simulink model "DualMotorElectricVehicle_full_Accel_full_Brake"  (R2023b)
settings: Solver=FixedStepAuto  StartTime=0.0  StopTime=300  FixedStep=0.01  RelTol=1e-3
values from neighbouring files (symbols this model uses):
  Af = 2.4    [DualMotorElectricVehicle.m]    (also in DualMotorElectricVehicle_Parameter.m)
  Cd = 0.24    [DualMotorElectricVehicle.m]    (also in DualMotorElectricVehicle_Parameter.m)
  eff_map_f = [ 81.3 81.3 82.2 82.0 81.5 81.2 80.4 79.3 80.1 76.8 74.3 73.5 72.0 71.6 70.0 71.1 ... (first row only)    [DualMotorElectricVehicle.m]    (also in DualMotorElectricVehicle_Parameter.m)
  eff_map_r = [ 36.6 36.6 36.6 36.6 36.6 36.6 36.6 36.6 36.6 36.6 36.6 36.6 36.6 36.6 36.6 36.6 36.6 36.6 36.6 36.6 36.6 36.6 36.6 36.6 36.6 36.6 36.6 36.6 36.6 36.6 36.6 36.6 36.6 36.6 36.6 36.6 36.6 36.6 36.6 36.6 36.6 ... (first row only)    [DualMotorElectricVehicle.m]    (also in DualMotorElectricVehicle_Parameter.m)
  eff_spd_f = [0 105 209 314 419 524 628 733 838 943 1047 1152 1257 1361]*30/pi    [DualMotorElectricVehicle.m]    (also in DualMotorElectricVehicle_Parameter.m)
  eff_spd_r = [0 300 500 700 900 1100 1300 1500 1700 1900 2100 2300 2500 2700 3000 3400 3800 4200 4600 5000 5400 5800 6000]    [DualMotorElectricVehicle.m]    (also in DualMotorElectricVehicle_Parameter.m)
  eff_trq_f = [0.0 13.6 27.1 40.7 54.2 67.8 81.4 94.9 108.5 122.0 135.6 149.2 162.7 176.3 189.8 203.4]    [DualMotorElectricVehicle.m]    (also in DualMotorElectricVehicle_Parameter.m)
  eff_trq_r = [0:5:200]*125/200    [DualMotorElectricVehicle.m]    (also in DualMotorElectricVehicle_Parameter.m)
  f_roll = 0.015    [DualMotorElectricVehicle.m]    (also in DualMotorElectricVehicle_Parameter.m)
  g = 9.81    [DualMotorElectricVehicle.m]    (also in DualMotorElectricVehicle_Parameter.m)
  G_final = 8    [DualMotorElectricVehicle.m]    (also in DualMotorElectricVehicle_Parameter.m)
  M_veh = 2000    [DualMotorElectricVehicle.m]    (also in DualMotorElectricVehicle_Parameter.m)
  Q_bat = 28    [DualMotorElectricVehicle.m]    (also in DualMotorElectricVehicle_Parameter.m)
  R_final = 4    [DualMotorElectricVehicle.m]    (also in DualMotorElectricVehicle_Parameter.m)
  R_int = 0.2811    [DualMotorElectricVehicle.m]    (also in DualMotorElectricVehicle_Parameter.m)
  r_tire = 0.35    [DualMotorElectricVehicle.m]    (also in DualMotorElectricVehicle_Parameter.m)
  rho = 1.16    [DualMotorElectricVehicle.m]    (also in DualMotorElectricVehicle_Parameter.m)
  SOC_init = 0.9    [DualMotorElectricVehicle.m]    (also in DualMotorElectricVehicle_Parameter.m = 0.8)
  SOC_min = 0.2    [DualMotorElectricVehicle.m]    (also in DualMotorElectricVehicle_Parameter.m = 0.4)
  tau_f = 0.05    [DualMotorElectricVehicle_Parameter.m]
  tau_m = 0.015    [DualMotorElectricVehicle_Parameter.m]
  theta = 0    [DualMotorElectricVehicle.m]    (also in DualMotorElectricVehicle_Parameter.m)
  Tm_max_spd_f = [0 300 419 524 628 733 838 943 1047 1152 1257 1361 1461 1561]*30/pi    [DualMotorElectricVehicle.m]    (also in DualMotorElectricVehicle_Parameter.m)
  Tm_max_spd_r = [0 1230 1300 1500:500:5500 5800 6000]    [DualMotorElectricVehicle.m]    (also in DualMotorElectricVehicle_Parameter.m)
  Tm_max_trq_f = [203 203 193 156 129 111 98 85 79 72 65 60 0 0]    [DualMotorElectricVehicle.m]    (also in DualMotorElectricVehicle_Parameter.m)
  Tm_max_trq_r = [125 125 117.53 101.86 76.39 61.12 50.93 43.65 38.20 33.95 30.56 27.78 0 0]    [DualMotorElectricVehicle.m]    (also in DualMotorElectricVehicle_Parameter.m)
  VOC_map = No_cell * [3.19, 3.40, 3.47, 3.59, 3.62, 3.65, 3.69, 3.74, 3.82, 3.89, 3.96]    [DualMotorElectricVehicle.m]    (also in DualMotorElectricVehicle_Parameter.m)
  VOC_SOC = [0, 0.1, 0.2, 0.3, 0.4, 0.5, 0.6 0.7, 0.8, 0.9, 1]    [DualMotorElectricVehicle.m]    (also in DualMotorElectricVehicle_Parameter.m)
  Vt_init = 311    [DualMotorElectricVehicle.m]    (also in DualMotorElectricVehicle_Parameter.m)
libraries: SignalEditorBlockLib x2
settings Model: Creator=김준현  LastModifiedBy=김준현

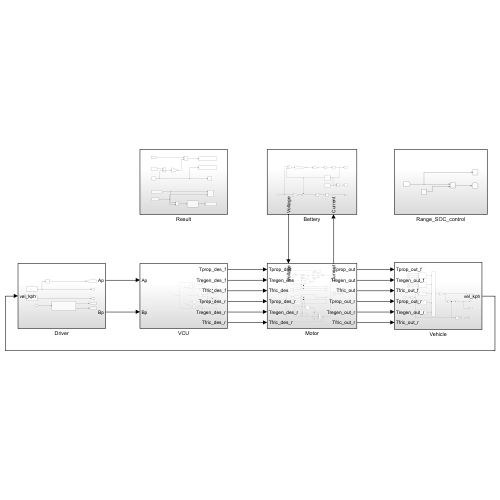
[thumbnail: Simulink's stored preview of the top-level diagram]
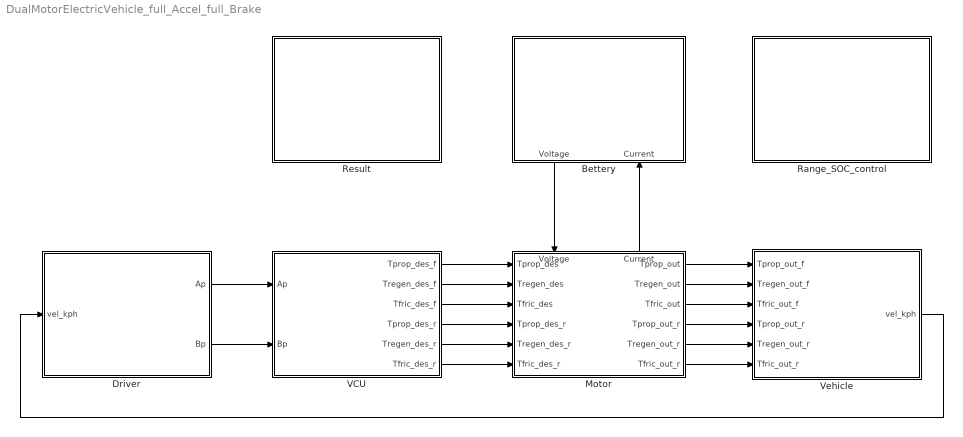
== system DualMotorElectricVehicle_full_Accel_full_Brake ==
  Bettery : Subsystem
      settings: PortSchema="{\"entries\":[{\"content\":{\"sides\":[{\"content\":{},\"type\":\"ConnectorPlacement.EquallySpacedRectSide\",\"uuid\":\"4f8bbb1a-fa5a-421b-ae69-e0b44ed86b01\"},{\"content\":{\"side\":\"RIGHT\"},\"type\":\"ConnectorPlacement.EquallySpacedRectSide\",\"uuid\":\"64d9ef76-34ca-4a4b-a58c-5ada3c393ba3\"},{\"content\":{\"side\":\"TOP\"},\"type\":\"ConnectorPlacement.EquallySpacedRectSide\",\"uuid\":\"8e5f7bf2-c6ce-4b8d-bfcf-b49871de395a\"},{\"content\":{\"connectorIds\":[\"Out1\",\"In1\"],\"side\":\"BOTTOM\"},\"type\":\"ConnectorPlacement.EquallySpacedRectSide\",\"uuid\":\"99b45dde-6c00-4863-951a-4b4ae2772398\"}]},\"type\":\"ConnectorPlacement.EquallySpacedConnector\",\"uuid\":\"2f749249-48ed-4409-ad27-f14061cdc912\"}],\"packageUris\":[\"http://schema.mathworks.com/mf0/Connector/R2020b\"],\"version\":\"1.0\"}"
  Driver : Subsystem
  Motor : Subsystem
      settings: PortSchema="{\"entries\":[{\"content\":{\"sides\":[{\"content\":{\"connectorIds\":[\"In1\",\"In2\",\"In3\",\"In4\",\"In5\",\"In6\"]},\"type\":\"ConnectorPlacement.EquallySpacedRectSide\",\"uuid\":\"a94dc67e-5088-4d58-a4ca-eb86600f42a3\"},{\"content\":{\"connectorIds\":[\"Out1\",\"Out2\",\"Out3\",\"Out4\",\"Out5\",\"Out6\"],\"side\":\"RIGHT\"},\"type\":\"ConnectorPlacement.EquallySpacedRectSide\",\"uuid\":\"bb581995-727b-4bbc-b281-e0daf5ac58fc\"},{\"content\":{\"connectorIds\":[\"In7\",\"Out7\"],\"side\":\"TOP\"},\"type\":\"ConnectorPlacement.EquallySpacedRectSide\",\"uuid\":\"7ea9d0e6-8443-414c-bafd-4c6fdb6eb2aa\"}]},\"type\":\"ConnectorPlacement.EquallySpacedConnector\",\"uuid\":\"c06b5305-48a4-41e7-b050-c7ca45c72c8b\"}],\"packageUris\":[\"http://schema.mathworks.com/mf0/Connector/R2020b\"],\"version\":\"1.0\"}"
  Range_SOC_control : Subsystem
  Result : Subsystem
  VCU : Subsystem
  Vehicle : Subsystem
  wires:
  Driver/1(Ap) -> VCU/1(Ap)
  Driver/2(Bp) -> VCU/2(Bp)
  VCU/1(Tprop_des_f) -> Motor/1(Tprop_des)
  VCU/2(Tregen_des_f) -> Motor/2(Tregen_des)
  VCU/3(Tfric_des_f) -> Motor/3(Tfric_des)
  Bettery/1(Voltage) -> Motor/7(Voltage)
  Motor/7(Current) -> Bettery/1(Current)
  Motor/1(Tprop_out) -> Vehicle/1(Tprop_out_f)
  Motor/2(Tregen_out) -> Vehicle/2(Tregen_out_f)
  Motor/3(Tfric_out) -> Vehicle/3(Tfric_out_f)
  Vehicle/1(vel_kph) -> Driver/1(vel_kph)
  VCU/4(Tprop_des_r) -> Motor/4(Tprop_des_r)
  VCU/5(Tregen_des_r) -> Motor/5(Tregen_des_r)
  VCU/6(Tfric_des_r) -> Motor/6(Tfric_des_r)
  Motor/4(Tprop_out_r) -> Vehicle/4(Tprop_out_r)
  Motor/5(Tregen_out_r) -> Vehicle/5(Tregen_out_r)
  Motor/6(Tfric_out_r) -> Vehicle/6(Tfric_out_r)

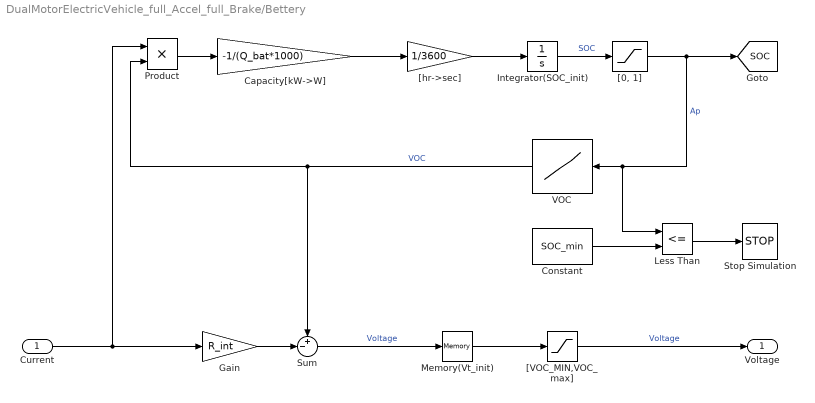
== system DualMotorElectricVehicle_full_Accel_full_Brake/Bettery ==
  Current : Inport
  Capacity[kW->W] : Gain  Gain=-1/(Q_bat*1000)
  Constant : Constant  Value=SOC_min
  Gain : Gain  Gain=R_int
  Integrator(SOC_init) : Integrator  InitialCondition=SOC_init
  Less Than : RelationalOperator  Operator=<=  OutDataTypeStr=boolean  RndMeth=Simplest  InputSameDT=off
  Memory(Vt_init) : Memory  InitialCondition=Vt_init
  Product : Product
  Stop Simulation : Stop
  Sum : Sum  Inputs=+-|
  VOC : Lookup_n-D  NumberOfTableDimensions=1  BreakpointsForDimension1=VOC_SOC  Table=VOC_map  InternalRulePriority=Speed  RndMeth=Simplest
  "[0, 1]" : Saturate  UpperLimit=1  LowerLimit=0
  "[VOC_MIN,VOC_max]" : Saturate  UpperLimit=max(VOC_map)  LowerLimit=min(VOC_map)
  "[hr->sec]" : Gain  Gain=1/3600
  Voltage : Outport
  tag scope: SOC=global
  wires:
  Current/1 -> Gain/1, Product/1
  VOC/1 -> Sum/1, Product/2  "VOC"
  Product/1 -> Capacity[kW->W]/1
  Capacity[kW->W]/1 -> "[hr->sec]"/1
  "[hr->sec]"/1 -> Integrator(SOC_init)/1
  Integrator(SOC_init)/1 -> "[0, 1]"/1  "SOC"
  Gain/1 -> Sum/2
  Sum/1 -> Memory(Vt_init)/1  "Voltage"
  "[VOC_MIN,VOC_max]"/1 -> Voltage/1  "Voltage"
  Memory(Vt_init)/1 -> "[VOC_MIN,VOC_max]"/1
  Less Than/1 -> Stop Simulation/1
  Constant/1 -> Less Than/2
  "[0, 1]"/1 -> [SOC], Less Than/1, VOC/1  "Ap"

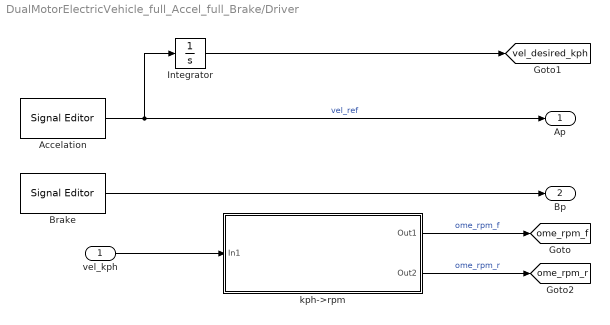
== system DualMotorElectricVehicle_full_Accel_full_Brake/Driver ==
  vel_kph : Inport
  Accelation : SignalEditorBlockLib/Signal Editor  FileName=AP.mat  ActiveScenario=Scenario  ActiveSignal=Step  IsBus=off  OutputBusObjectStr=Bus: BusObject  SampleTime=0  Interpolate=off  ZeroCross=off  OutputAfterFinalValue=Setting to zero  Unit=inherit  PreserveSignalName=on  ApplySigPropsToAllScenarios=on  ApplySigPropsToAllSignals=off
  Brake : SignalEditorBlockLib/Signal Editor  FileName=BP.mat  ActiveScenario=Scenario  ActiveSignal=Signal 1  IsBus=off  OutputBusObjectStr=Bus: BusObject  SampleTime=0  Interpolate=off  ZeroCross=off  OutputAfterFinalValue=Setting to zero  Unit=inherit  PreserveSignalName=on  ApplySigPropsToAllScenarios=on  ApplySigPropsToAllSignals=off
  Integrator : Integrator
  kph->rpm : Subsystem
  Ap : Outport
  Bp : Outport  Port=2
  tag scope: ome_rpm_f=global, ome_rpm_r=global, vel_desired_kph=global
  wires:
  kph->rpm/1(Out1) -> [ome_rpm_f]  "ome_rpm_f"
  vel_kph/1 -> kph->rpm/1(In1)
  Accelation/1 -> Ap/1, Integrator/1  "vel_ref"
  Integrator/1 -> [vel_desired_kph]
  Brake/1 -> Bp/1
  kph->rpm/2(Out2) -> [ome_rpm_r]  "ome_rpm_r"

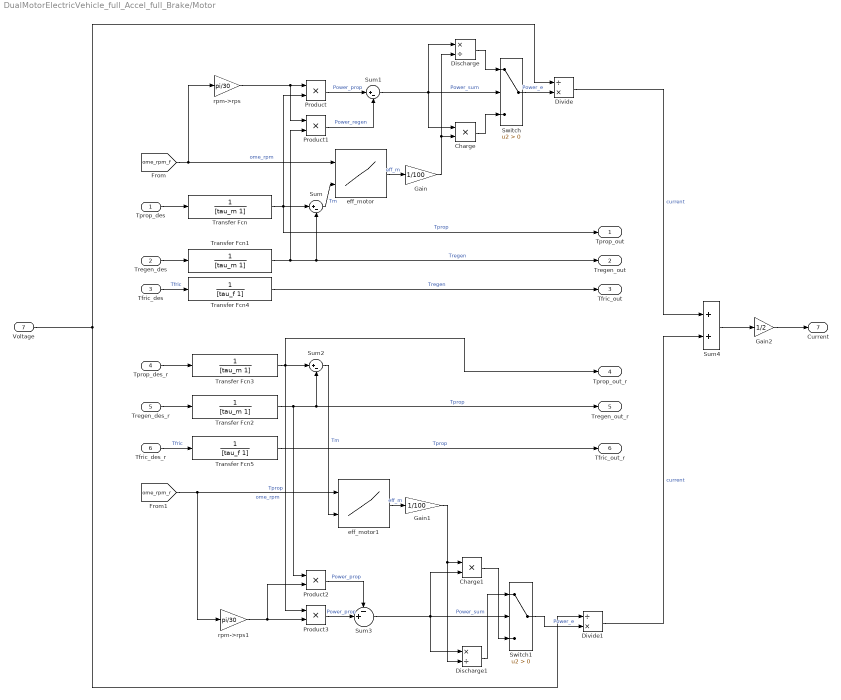
== system DualMotorElectricVehicle_full_Accel_full_Brake/Motor ==
  Tprop_des : Inport
  Tregen_des : Inport  Port=2
  Tfric_des : Inport  Port=3
  Tprop_des_r : Inport  Port=4
  Tregen_des_r : Inport  Port=5
  Tfric_des_r : Inport  Port=6
  Voltage : Inport  Port=7
  Charge : Product
  Charge1 : Product
  Discharge : Product  Inputs=*/
  Discharge1 : Product  Inputs=*/
  Divide : Product  Inputs=/*
  Divide1 : Product  Inputs=/*
  Gain : Gain  Gain=1/100
  Gain1 : Gain  Gain=1/100
  Gain2 : Gain  Gain=1/2
  Product{,1..3} (4 alike) : Product
  Sum : Sum  Inputs=|+-
  Sum1 : Sum  Inputs=|+-
  Sum2 : Sum  Inputs=|+-
  Sum3 : Sum  Inputs=-+|
  Sum4 : Sum
  Switch : Switch  Criteria=u2 > Threshold  SaturateOnIntegerOverflow=off  InputSameDT=off
  Switch1 : Switch  Criteria=u2 > Threshold  SaturateOnIntegerOverflow=off  InputSameDT=off
  Transfer Fcn{,1..3} (4 alike) : TransferFcn  Denominator=[tau_m 1]
  Transfer Fcn4 : TransferFcn  Denominator=[tau_f 1]
  Transfer Fcn5 : TransferFcn  Denominator=[tau_f 1]
  eff_motor : Lookup_n-D  BreakpointsForDimension1=eff_spd_f  BreakpointsForDimension2=eff_trq_f  Table=eff_map_f  InternalRulePriority=Speed  RndMeth=Simplest
      settings: InputPortMap=u0,u1
  eff_motor1 : Lookup_n-D  BreakpointsForDimension1=eff_spd_r  BreakpointsForDimension2=eff_trq_r  Table=eff_map_r  InternalRulePriority=Speed  RndMeth=Simplest
      settings: InputPortMap=u0,u1
  rpm->rps : Gain  Gain=pi/30
  rpm->rps1 : Gain  Gain=pi/30
  Tprop_out : Outport
  Tregen_out : Outport  Port=2
  Tfric_out : Outport  Port=3
  Tprop_out_r : Outport  Port=4
  Tregen_out_r : Outport  Port=5
  Tfric_out_r : Outport  Port=6
  Current : Outport  Port=7
  wires:
  Tprop_des/1 -> Transfer Fcn/1
  Transfer Fcn/1 -> Tprop_out/1, Product/2, Sum/1  "Tprop"
  Transfer Fcn1/1 -> Product1/2, Sum/2, Tregen_out/1  "Tregen"
  Tregen_des/1 -> Transfer Fcn1/1
  Sum/1 -> eff_motor/2  "Tm"
  [ome_rpm_f] -> rpm->rps/1, eff_motor/1  "ome_rpm"
  rpm->rps/1 -> Product1/1, Product/1
  Product/1 -> Sum1/1  "Power_prop"
  Product1/1 -> Sum1/2  "Power_regen"
  Sum1/1 -> Charge/1, Discharge/1, Switch/2  "Power_sum"
  Charge/1 -> Switch/3
  Discharge/1 -> Switch/1
  Tfric_des/1 -> Transfer Fcn4/1  "Tfric"
  Switch/1 -> Divide/2  "Power_e"
  Voltage/1 -> Divide1/1, Divide/1
  Divide/1 -> Sum4/1  "current"
  Tfric_des_r/1 -> Transfer Fcn5/1  "Tfric"
  Tregen_des_r/1 -> Transfer Fcn2/1
  Transfer Fcn2/1 -> Product2/1, Tregen_out_r/1, Sum2/2  "Tprop"
  Transfer Fcn3/1 -> Product3/1, Tprop_out_r/1, Sum2/1  "Tprop"
  Tprop_des_r/1 -> Transfer Fcn3/1
  [ome_rpm_r] -> rpm->rps1/1, eff_motor1/1  "ome_rpm"
  Sum2/1 -> eff_motor1/2  "Tm"
  Charge1/1 -> Switch1/3
  rpm->rps1/1 -> Product2/2, Product3/2
  Product3/1 -> Sum3/2  "Power_prop"
  Product2/1 -> Sum3/1  "Power_prop"
  Sum3/1 -> Discharge1/1, Charge1/2, Switch1/2  "Power_sum"
  Discharge1/1 -> Switch1/1
  Switch1/1 -> Divide1/2  "Power_e"
  Divide1/1 -> Sum4/2  "current"
  eff_motor/1 -> Gain/1  "eff_m"
  Gain/1 -> Charge/2, Discharge/2
  eff_motor1/1 -> Gain1/1  "eff_m"
  Gain1/1 -> Discharge1/2, Charge1/1
  Gain2/1 -> Current/1
  Sum4/1 -> Gain2/1
  Transfer Fcn4/1 -> Tfric_out/1  "Tregen"
  Transfer Fcn5/1 -> Tfric_out_r/1  "Tprop"

== system DualMotorElectricVehicle_full_Accel_full_Brake/Range_SOC_control ==
  Constant : Constant  Value=0.4
  Less Than : RelationalOperator  Operator=<=  OutDataTypeStr=boolean  RndMeth=Simplest  InputSameDT=off
  Scope : Scope
  Stop Simulation : Stop
  wires:
  Less Than/1 -> Stop Simulation/1
  Constant/1 -> Less Than/2
  [SOC] -> Scope/1, Less Than/1

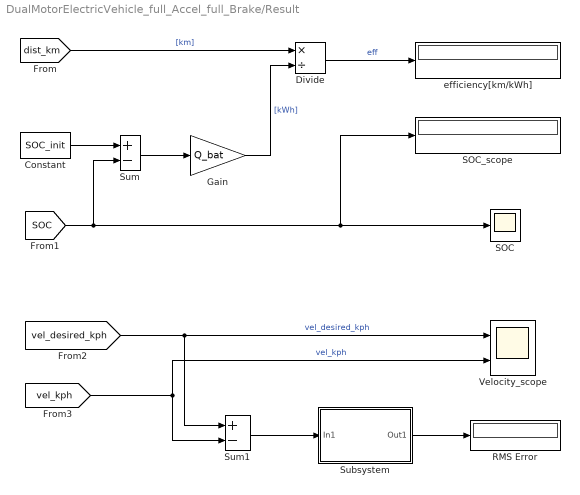
== system DualMotorElectricVehicle_full_Accel_full_Brake/Result ==
  Constant : Constant  Value=SOC_init
  Divide : Product  Inputs=*/
  Gain : Gain  Gain=Q_bat
  RMS Error : Display
  SOC : Scope
  SOC_scope : Display
  Subsystem : Subsystem
  Sum : Sum  Inputs=+-
  Sum1 : Sum  Inputs=+-
  Velocity_scope : Scope  NumInputPorts=2
  efficiency[km/kWh] : Display
  wires:
  Constant/1 -> Sum/1
  Sum/1 -> Gain/1
  [dist_km] -> Divide/1  "[km]"
  Gain/1 -> Divide/2  "[kWh]"
  Divide/1 -> efficiency[km/kWh]/1  "eff"
  [SOC] -> SOC_scope/1, SOC/1, Sum/2
  [vel_desired_kph] -> Sum1/1, Velocity_scope/1  "vel_desired_kph"
  [vel_kph] -> Sum1/2, Velocity_scope/2  "vel_kph"
  Subsystem/1(Out1) -> RMS Error/1
  Sum1/1 -> Subsystem/1(In1)

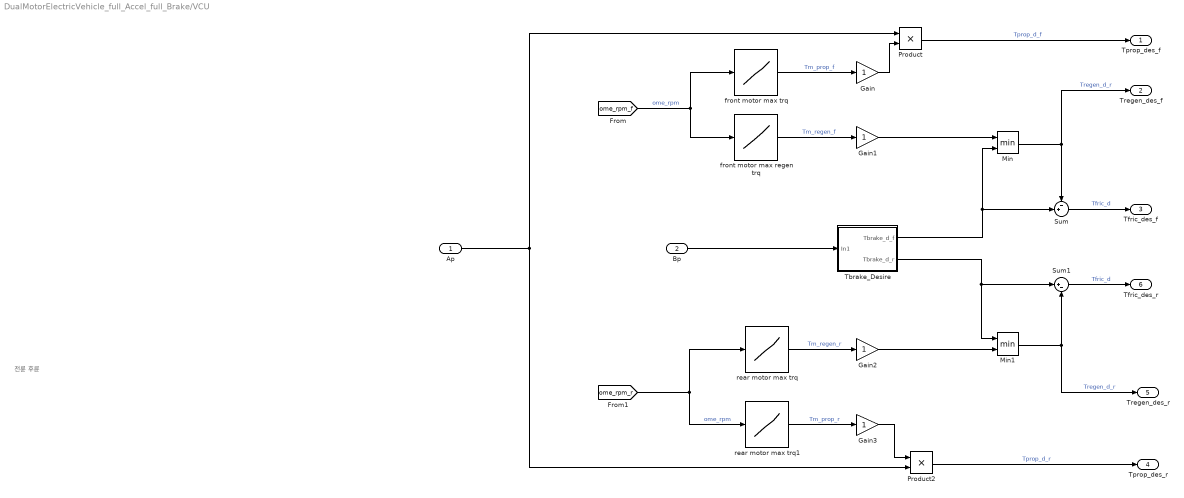
== system DualMotorElectricVehicle_full_Accel_full_Brake/VCU ==
  note: 전륜 후륜
  Ap : Inport
  Bp : Inport  Port=2
  Gain{,1..3} (4 alike) : Gain
  Min : MinMax  Inputs=2
  Min1 : MinMax  Inputs=2
  Product : Product
  Product2 : Product
  Sum : Sum  Inputs=-+|
  Sum1 : Sum  Inputs=|+-
  Tbrake_Desire : Subsystem
  front motor max regen trq : Lookup_n-D  NumberOfTableDimensions=1  BreakpointsForDimension1=Tm_max_spd_f  Table=Tm_max_trq_f  InternalRulePriority=Speed  RndMeth=Simplest
  front motor max trq : Lookup_n-D  NumberOfTableDimensions=1  BreakpointsForDimension1=Tm_max_spd_f  Table=Tm_max_trq_f  InternalRulePriority=Speed  RndMeth=Simplest
  rear motor max trq : Lookup_n-D  NumberOfTableDimensions=1  BreakpointsForDimension1=Tm_max_spd_r  Table=Tm_max_trq_r  InternalRulePriority=Speed  RndMeth=Simplest
  rear motor max trq1 : Lookup_n-D  NumberOfTableDimensions=1  BreakpointsForDimension1=Tm_max_spd_r  Table=Tm_max_trq_r  InternalRulePriority=Speed  RndMeth=Simplest
  Tprop_des_f : Outport
  Tregen_des_f : Outport  Port=2
  Tfric_des_f : Outport  Port=3
  Tprop_des_r : Outport  Port=4
  Tregen_des_r : Outport  Port=5
  Tfric_des_r : Outport  Port=6
  wires:
  Ap/1 -> Product2/2, Product/1
  [ome_rpm_f] -> front motor max regen trq/1, front motor max trq/1  "ome_rpm"
  front motor max trq/1 -> Gain/1  "Tm_prop_f"
  front motor max regen trq/1 -> Gain1/1  "Tm_regen_f"
  Gain/1 -> Product/2
  Product/1 -> Tprop_des_f/1  "Tprop_d_f"
  Gain1/1 -> Min/1
  Min/1 -> Sum/1, Tregen_des_f/1  "Tregen_d_r"
  Sum/1 -> Tfric_des_f/1  "Tfric_d"
  Bp/1 -> Tbrake_Desire/1(In1)
  [ome_rpm_r] -> rear motor max trq1/1, rear motor max trq/1  "ome_rpm"
  rear motor max trq/1 -> Gain2/1  "Tm_regen_r"
  rear motor max trq1/1 -> Gain3/1  "Tm_prop_r"
  Gain2/1 -> Min1/2
  Tbrake_Desire/1(Tbrake_d_f) -> Sum/2, Min/2
  Gain3/1 -> Product2/1
  Product2/1 -> Tprop_des_r/1  "Tprop_d_r"
  Sum1/1 -> Tfric_des_r/1  "Tfric_d"
  Min1/1 -> Tregen_des_r/1, Sum1/2  "Tregen_d_r"
  Tbrake_Desire/2(Tbrake_d_r) -> Min1/1, Sum1/1

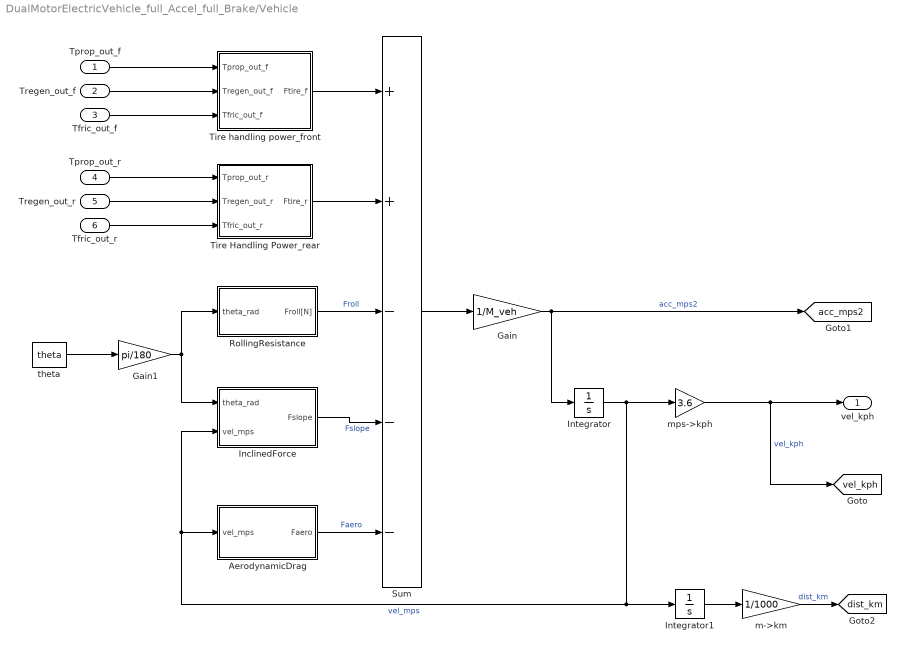
== system DualMotorElectricVehicle_full_Accel_full_Brake/Vehicle ==
  Tprop_out_f : Inport
  Tregen_out_f : Inport  Port=2
  Tfric_out_f : Inport  Port=3
  Tprop_out_r : Inport  Port=4
  Tregen_out_r : Inport  Port=5
  Tfric_out_r : Inport  Port=6
  AerodynamicDrag : Subsystem
  Gain : Gain  Gain=1/M_veh
  Gain1 : Gain  Gain=pi/180
  InclinedForce : Subsystem
  Integrator : Integrator
  Integrator1 : Integrator
  RollingResistance : Subsystem
  Sum : Sum  Inputs=++---
  Tire Handling Power_rear : Subsystem
  Tire handling power_front : Subsystem
  m->km : Gain  Gain=1/1000
  mps->kph : Gain  Gain=3.6
  theta : Constant  Value=theta
  vel_kph : Outport
  tag scope: acc_mps2=global, dist_km=global, vel_kph=global
  wires:
  Tprop_out_f/1 -> Tire handling power_front/1(Tprop_out_f)
  Tregen_out_f/1 -> Tire handling power_front/2(Tregen_out_f)
  Tfric_out_f/1 -> Tire handling power_front/3(Tfric_out_f)
  Tire handling power_front/1(Ftire_f) -> Sum/1
  Integrator/1 -> mps->kph/1, Integrator1/1, InclinedForce/2(vel_mps), AerodynamicDrag/1(vel_mps)  "vel_mps"
  Sum/1 -> Gain/1
  Gain/1 -> Integrator/1, [acc_mps2]  "acc_mps2"
  mps->kph/1 -> vel_kph/1, [vel_kph]  "vel_kph"
  Integrator1/1 -> m->km/1
  m->km/1 -> [dist_km]  "dist_km"
  theta/1 -> Gain1/1
  Gain1/1 -> InclinedForce/1(theta_rad), RollingResistance/1(theta_rad)
  InclinedForce/1(Fslope) -> Sum/4  "Fslope"
  AerodynamicDrag/1(Faero) -> Sum/5  "Faero"
  Tprop_out_r/1 -> Tire Handling Power_rear/1(Tprop_out_r)
  Tregen_out_r/1 -> Tire Handling Power_rear/2(Tregen_out_r)
  Tfric_out_r/1 -> Tire Handling Power_rear/3(Tfric_out_r)
  Tire Handling Power_rear/1(Ftire_r) -> Sum/2
  RollingResistance/1(Froll[N]) -> Sum/3  "Froll"

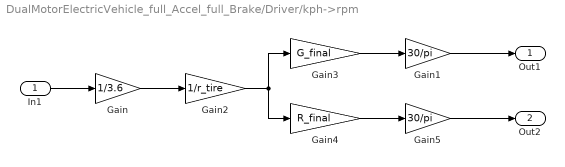
== system DualMotorElectricVehicle_full_Accel_full_Brake/Driver/kph->rpm ==
  In1 : Inport
  Gain : Gain  Gain=1/3.6
  Gain1 : Gain  Gain=30/pi
  Gain2 : Gain  Gain=1/r_tire
  Gain3 : Gain  Gain=G_final
  Gain4 : Gain  Gain=R_final
  Gain5 : Gain  Gain=30/pi
  Out1 : Outport
  Out2 : Outport  Port=2
  wires:
  Gain/1 -> Gain2/1
  In1/1 -> Gain/1
  Gain3/1 -> Gain1/1
  Gain2/1 -> Gain4/1, Gain3/1
  Gain1/1 -> Out1/1
  Gain4/1 -> Gain5/1
  Gain5/1 -> Out2/1

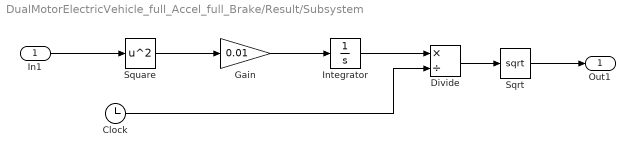
== system DualMotorElectricVehicle_full_Accel_full_Brake/Result/Subsystem ==
  In1 : Inport
  Clock : Clock
  Divide : Product  Inputs=*/
  Gain : Gain  Gain=0.01
  Integrator : Integrator
  Sqrt : Sqrt
  Square : Math  Operator=square
  Out1 : Outport
  wires:
  Clock/1 -> Divide/2
  Integrator/1 -> Divide/1
  Gain/1 -> Integrator/1
  Square/1 -> Gain/1
  Divide/1 -> Sqrt/1
  Sqrt/1 -> Out1/1
  In1/1 -> Square/1

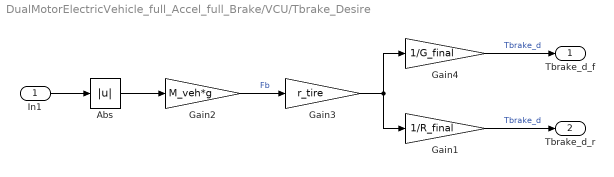
== system DualMotorElectricVehicle_full_Accel_full_Brake/VCU/Tbrake_Desire ==
  In1 : Inport
  Abs : Abs  SaturateOnIntegerOverflow=off
  Gain1 : Gain  Gain=1/R_final
  Gain2 : Gain  Gain=M_veh*g
  Gain3 : Gain  Gain=r_tire
  Gain4 : Gain  Gain=1/G_final
  Tbrake_d_f : Outport
  Tbrake_d_r : Outport  Port=2
  wires:
  Gain3/1 -> Gain4/1, Gain1/1
  Gain2/1 -> Gain3/1  "Fb"
  Gain4/1 -> Tbrake_d_f/1  "Tbrake_d"
  Abs/1 -> Gain2/1
  In1/1 -> Abs/1
  Gain1/1 -> Tbrake_d_r/1  "Tbrake_d"

== system DualMotorElectricVehicle_full_Accel_full_Brake/Vehicle/AerodynamicDrag ==
  vel_mps : Inport
  Interpreted MATLAB Function : MATLABFcn  MATLABFcn=1/2*rho*Cd*Af*u(1)^2
  Faero : Outport
  wires:
  vel_mps/1 -> Interpreted MATLAB Function/1
  Interpreted MATLAB Function/1 -> Faero/1

== system DualMotorElectricVehicle_full_Accel_full_Brake/Vehicle/InclinedForce ==
  theta_rad : Inport
  vel_mps : Inport  Port=2
  Interpreted MATLAB Function : MATLABFcn  MATLABFcn=M_veh*9.81*sin(u(1)*pi/180)
  Product : Product
  "[-1 1]" : Saturate  UpperLimit=1  LowerLimit=-1
  Fslope : Outport
  wires:
  theta_rad/1 -> Interpreted MATLAB Function/1
  Interpreted MATLAB Function/1 -> Product/1
  Product/1 -> Fslope/1
  vel_mps/1 -> "[-1 1]"/1
  "[-1 1]"/1 -> Product/2

== system DualMotorElectricVehicle_full_Accel_full_Brake/Vehicle/RollingResistance ==
  theta_rad : Inport
  Interpreted MATLAB Function : MATLABFcn  MATLABFcn=f_roll*M_veh*9.81*cos(u(1)*pi/180)
  Froll[N] : Outport
  wires:
  theta_rad/1 -> Interpreted MATLAB Function/1
  Interpreted MATLAB Function/1 -> Froll[N]/1

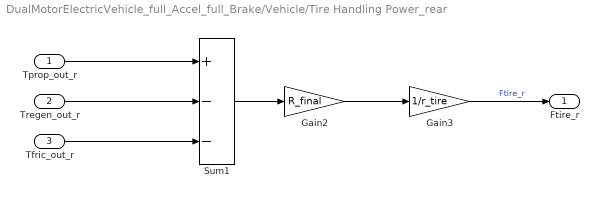
== system DualMotorElectricVehicle_full_Accel_full_Brake/Vehicle/Tire Handling Power_rear ==
  Tprop_out_r : Inport
  Tregen_out_r : Inport  Port=2
  Tfric_out_r : Inport  Port=3
  Gain2 : Gain  Gain=R_final
  Gain3 : Gain  Gain=1/r_tire
  Sum1 : Sum  Inputs=+--
  Ftire_r : Outport
  wires:
  Tregen_out_r/1 -> Sum1/2
  Tfric_out_r/1 -> Sum1/3
  Gain3/1 -> Ftire_r/1  "Ftire_r"
  Sum1/1 -> Gain2/1
  Gain2/1 -> Gain3/1
  Tprop_out_r/1 -> Sum1/1

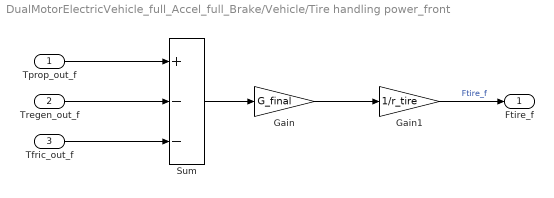
== system DualMotorElectricVehicle_full_Accel_full_Brake/Vehicle/Tire handling power_front ==
  Tprop_out_f : Inport
  Tregen_out_f : Inport  Port=2
  Tfric_out_f : Inport  Port=3
  Gain : Gain  Gain=G_final
  Gain1 : Gain  Gain=1/r_tire
  Sum : Sum  Inputs=+--
  Ftire_f : Outport
  wires:
  Tprop_out_f/1 -> Sum/1
  Tregen_out_f/1 -> Sum/2
  Tfric_out_f/1 -> Sum/3
  Sum/1 -> Gain/1
  Gain/1 -> Gain1/1
  Gain1/1 -> Ftire_f/1  "Ftire_f"
